simulink model "sampleModel2054_4_sub"  (R2023a)
settings: Solver=VariableStepAuto  StartTime=0.0  StopTime=10.0  RelTol=1e-3
libraries: hdlsllib x5, simulink x2
settings Model: Creator=user1  LastModifiedBy=user1

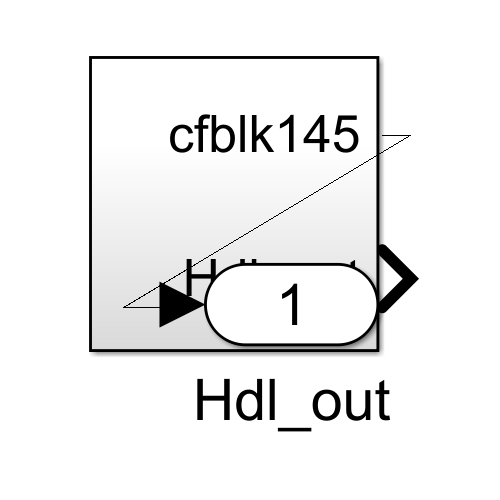
[thumbnail: Simulink's stored preview of the top-level diagram]
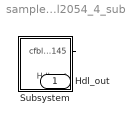
== system sampleModel2054_4_sub ==
  Subsystem : Subsystem
  Hdl_out : Outport  OutDataTypeStr=uint8
  wires:
  Subsystem/1(cfblk145) -> Hdl_out/1

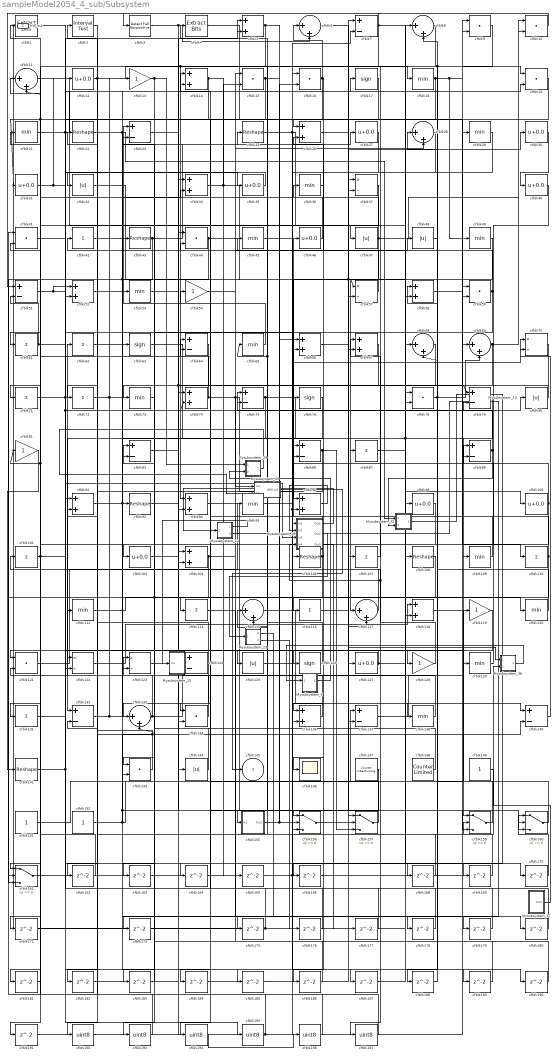
== system sampleModel2054_4_sub/Subsystem ==
  Mysubsystem_12 : Subsystem  TreatAsAtomicUnit=on  RTWFcnName=Mysubsystem_12
      settings: RTWFcnNameOpts=User specified  RTWFileNameOpts=Use function name
  Mysubsystem_13 : Subsystem  TreatAsAtomicUnit=on  RTWFcnName=Mysubsystem_13
      settings: RTWFcnNameOpts=User specified  RTWFileNameOpts=Use function name
  Mysubsystem_15 : Subsystem  TreatAsAtomicUnit=on  RTWFcnName=Mysubsystem_15
      settings: RTWFcnNameOpts=User specified  RTWFileNameOpts=Use function name
  Mysubsystem_19 : Subsystem  TreatAsAtomicUnit=on  RTWFcnName=Mysubsystem_19
      settings: RTWFcnNameOpts=User specified  RTWFileNameOpts=Use function name
  Mysubsystem_23 : Subsystem  TreatAsAtomicUnit=on  RTWFcnName=Mysubsystem_23
      settings: RTWFcnNameOpts=User specified  RTWFileNameOpts=Use function name
  Mysubsystem_24 : Subsystem  TreatAsAtomicUnit=on  RTWFcnName=Mysubsystem_24
      settings: RTWFcnNameOpts=User specified  RTWFileNameOpts=Use function name
  Mysubsystem_25 : Subsystem  TreatAsAtomicUnit=on  RTWFcnName=Mysubsystem_25
      settings: RTWFcnNameOpts=User specified  RTWFileNameOpts=Use function name
  Mysubsystem_32 : Subsystem  TreatAsAtomicUnit=on  RTWFcnName=Mysubsystem_32
      settings: RTWFcnNameOpts=User specified  RTWFileNameOpts=Use function name
  Mysubsystem_36 : Subsystem  TreatAsAtomicUnit=on  RTWFcnName=Mysubsystem_36
      settings: RTWFcnNameOpts=User specified  RTWFileNameOpts=Use function name
  Mysubsystem_37 : Subsystem  TreatAsAtomicUnit=on  RTWFcnName=Mysubsystem_37
      settings: RTWFcnNameOpts=User specified  RTWFileNameOpts=Use function name
  Mysubsystem_6 : Subsystem  TreatAsAtomicUnit=on  RTWFcnName=Mysubsystem_6
      settings: RTWFcnNameOpts=User specified  RTWFileNameOpts=Use function name
  cfblk1 : simulink/Logic and Bit Operations/Extract Bits  bitsToExtract=Upper half  numBits=8  bitIdxRange=[0 7]  outScalingMode=Preserve fixed-point scaling
      settings: LibrarySourceBlock=|
      | hdlsllib/Logic and Bit
      | Operations/Extract Bits
  cfblk{9..10,15..16,20,41,44,59,78,121,134,143} (12 alike) : DotProduct  OutDataTypeStr=uint8
  cfblk{12,27,30..31,35,40,46,98,100,103,127} (11 alike) : Bias  Bias=0.0  SaturateOnIntegerOverflow=off
  cfblk{42,61..62,71..72,87,101,107,110,114,116,131} (12 alike) : Sum  Inputs=+  OutDataTypeStr=uint8
  cfblk{5,14,26,34,52,58,66..67,74,92,94,96,104,118,136} (15 alike) : Sum  OutDataTypeStr=uint8
  cfblk{22,25,43,93,106,108,141} (7 alike) : Reshape
  cfblk{18,21,29,36,45,49,53,65,73,95,109,112,120,129,138} (15 alike) : MinMax  OutDataTypeStr=uint8
  cfblk{6,8,11,28,68..69,115,117,133} (9 alike) : Sum  Inputs=|++  OutDataTypeStr=uint8
  cfblk{13,54,81,119,128} (5 alike) : Gain  OutDataTypeStr=uint8
  cfblk{37,57,70,122..123} (5 alike) : Product  Inputs=*/  OutDataTypeStr=uint8  RndMeth=Zero  SaturateOnIntegerOverflow=on
  cfblk{7,23,51,64,75,79,83,86,89,124,132,137,140} (13 alike) : Sum  Inputs=+-  OutDataTypeStr=uint8
  cfblk{32,47..48,80,125,144} (6 alike) : Abs  OutDataTypeStr=uint8  SaturateOnIntegerOverflow=off
  cfblk{17,63,76,126} (4 alike) : Signum
  cfblk146 : Scope
  cfblk147 : hdlsllib/Sources/Counter Free-Running  NumBits=16  tsamp=-1
  cfblk148 : hdlsllib/Sources/Counter Limited  uplimit=7  tsamp=-1
  cfblk149 : Constant  OutDataTypeStr=uint8  SampleTime=-1
  cfblk151 : Constant  OutDataTypeStr=uint8  SampleTime=-1
  cfblk152 : Constant  OutDataTypeStr=uint8  SampleTime=-1
  cfblk155 : Subsystem
      settings: LibrarySourceBlock=|
      | hdlsllib/Ports &
      | Subsystems/Subsystem
  cfblk{156..157,159..161} (5 alike) : Switch  OutDataTypeStr=uint8  SaturateOnIntegerOverflow=off  InputSameDT=off
  cfblk{162..166,168..171,173,175..191} (27 alike) : Delay  SampleTime=1
  cfblk{192..197} (6 alike) : DataTypeConversion  OutDataTypeStr=uint8  SaturateOnIntegerOverflow=off  RndMeth=Floor
  cfblk2 : hdlsllib/Logic and Bit Operations/Interval Test  IntervalClosedRight=on  uplimit=0.5  IntervalClosedLeft=on  lowlimit=-0.5  OutDataTypeStr=uint8
  cfblk3 : hdlsllib/Logic and Bit Operations/Detect Fall Nonpositive  vinit=0  OutDataTypeStr=uint8
  cfblk4 : simulink/Logic and Bit Operations/Extract Bits  bitsToExtract=Upper half  numBits=8  bitIdxRange=[0 7]  outScalingMode=Preserve fixed-point scaling
      settings: LibrarySourceBlock=|
      | hdlsllib/Logic and Bit
      | Operations/Extract Bits
  cfblk145 : Outport  OutDataTypeStr=uint8  VectorParamsAs1DForOutWhenUnconnected=off
  Hdl_out : Outport  Port=2  OutDataTypeStr=uint8
  wires:
  cfblk5/1 -> cfblk66/1, cfblk61/1, cfblk94/1
  cfblk127/1 -> cfblk80/1, cfblk121/1
  cfblk79/1 -> cfblk159/1
  cfblk72/1 -> cfblk190/1, cfblk63/1
  cfblk51/1 -> cfblk170/1, cfblk52/1
  cfblk94/1 -> cfblk156/1
  cfblk70/1 -> cfblk114/1
  cfblk43/1 -> cfblk161/2, cfblk25/1
  cfblk144/1 -> cfblk83/1
  cfblk15/1 -> cfblk156/2, cfblk191/1, cfblk31/1
  cfblk86/1 -> cfblk162/1, cfblk157/3
  cfblk76/1 -> cfblk132/1
  cfblk57/1 -> cfblk42/1
  cfblk110/1 -> cfblk122/2, cfblk46/1
  cfblk41/1 -> cfblk195/1
  cfblk122/1 -> cfblk118/1
  cfblk81/1 -> cfblk141/1
  cfblk62/1 -> cfblk27/1
  cfblk117/1 -> cfblk64/1
  cfblk65/1 -> cfblk23/1
  cfblk44/1 -> cfblk183/1, cfblk57/2, cfblk98/1
  cfblk49/1 -> cfblk96/1
  cfblk59/1 -> cfblk36/1, cfblk133/1
  cfblk16/1 -> cfblk182/1, cfblk146/1, cfblk6/1
  cfblk10/1 -> cfblk51/1
  cfblk3/1 -> cfblk117/2, cfblk6/2
  cfblk30/1 -> cfblk40/1
  cfblk148/1 -> cfblk53/1
  cfblk149/1 -> cfblk159/2
  cfblk13/1 -> cfblk133/2, Mysubsystem_24/1(In1)
  cfblk20/1 -> cfblk125/1
  cfblk63/1 -> cfblk108/1
  cfblk45/1 -> cfblk47/1
  cfblk112/1 -> cfblk120/1
  cfblk151/1 -> cfblk137/1
  cfblk78/1 -> cfblk178/1, cfblk69/2
  cfblk34/1 -> cfblk15/2, cfblk117/1
  cfblk83/1 -> cfblk124/1
  cfblk161/1 -> cfblk37/2, cfblk16/1
  cfblk136/1 -> cfblk62/1
  cfblk32/1 -> cfblk127/1
  cfblk42/1 -> cfblk168/1, cfblk160/2
  cfblk61/1 -> cfblk20/2, cfblk51/2
  cfblk52/1 -> cfblk87/1
  cfblk126/1 -> cfblk4/1
  cfblk159/1 -> cfblk119/1
  cfblk25/1 -> cfblk140/1, cfblk78/1
  cfblk95/1 -> cfblk7/2
  cfblk98/1 -> cfblk155/1(In1)
  cfblk128/1 -> Mysubsystem_19/4(In4), cfblk101/1
  cfblk106/1 -> cfblk44/2, cfblk143/1
  cfblk26/1 -> cfblk159/3
  cfblk73/1 -> cfblk43/1
  cfblk11/1 -> cfblk78/2
  cfblk121/1 -> cfblk95/1
  cfblk119/1 -> cfblk131/1
  cfblk8/1 -> cfblk115/2
  cfblk74/1 -> cfblk21/1, cfblk106/1, Mysubsystem_25/1(In1)
  cfblk160/1 -> cfblk58/1
  cfblk18/1 -> cfblk71/1, cfblk20/1, cfblk49/1
  cfblk138/1 -> cfblk75/1
  cfblk64/1 -> cfblk104/2
  cfblk157/1 -> cfblk54/1
  cfblk53/1 -> cfblk160/3, cfblk79/1
  cfblk31/1 -> cfblk189/1, cfblk12/1
  cfblk22/1 -> cfblk179/1, cfblk57/1, Mysubsystem_32/1(In1)
  cfblk47/1 -> cfblk26/2, cfblk126/1, cfblk10/1
  cfblk124/1 -> cfblk163/1, cfblk92/2
  cfblk75/1 -> cfblk134/1, cfblk107/1
  cfblk134/1 -> cfblk123/1
  cfblk116/1 -> cfblk128/1
  cfblk118/1 -> cfblk29/1
  cfblk104/1 -> cfblk48/1, cfblk193/1, cfblk161/3
  cfblk101/1 -> cfblk171/1, Mysubsystem_19/3(In3)
  cfblk100/1 -> cfblk161/1, cfblk86/2
  cfblk132/1 -> cfblk13/1, cfblk34/2
  cfblk27/1 -> cfblk137/2
  cfblk155/1(Out1) -> cfblk16/2, cfblk70/1
  cfblk129/1 -> cfblk89/1
  cfblk21/1 -> cfblk66/2, cfblk26/1, cfblk17/1
  cfblk152/1 -> cfblk140/2, cfblk59/1
  cfblk89/1 -> cfblk75/2, Mysubsystem_32/2(In2)
  cfblk103/1 -> cfblk76/1
  cfblk4/1 -> cfblk59/2
  cfblk29/1 -> cfblk96/2, Mysubsystem_19/1(In1)
  cfblk137/1 -> cfblk9/1
  cfblk69/1 -> cfblk116/1, cfblk10/2
  cfblk54/1 -> cfblk28/2
  cfblk40/1 -> cfblk109/1
  cfblk12/1 -> cfblk18/1, cfblk72/1
  cfblk156/1 -> cfblk30/1
  cfblk93/1 -> cfblk79/2
  cfblk120/1 -> cfblk8/2
  cfblk23/1 -> cfblk74/1
  cfblk35/1 -> cfblk32/1
  cfblk68/1 -> cfblk103/1
  cfblk80/1 -> cfblk73/1
  cfblk1/1 -> cfblk35/1
  cfblk9/1 -> cfblk197/1, cfblk68/2
  cfblk14/1 -> cfblk165/1, cfblk112/1
  cfblk133/1 -> cfblk118/2, cfblk81/1, cfblk11/2
  cfblk46/1 -> cfblk11/1
  cfblk67/1 -> cfblk123/2
  cfblk143/1 -> cfblk122/1, cfblk22/1
  cfblk107/1 -> cfblk67/1
  cfblk71/1 -> cfblk5/2, cfblk74/2, cfblk129/1
  cfblk58/1 -> cfblk110/1
  cfblk109/1 -> cfblk45/1, cfblk65/1
  cfblk115/1 -> cfblk138/1
  cfblk140/1 -> cfblk70/2
  cfblk28/1 -> cfblk136/1
  cfblk7/1 -> cfblk3/1, cfblk134/2, cfblk89/2, cfblk100/1
  cfblk92/1 -> cfblk14/1, cfblk93/1
  cfblk6/1 -> cfblk37/1
  cfblk141/1 -> cfblk185/1, cfblk52/2
  cfblk108/1 -> cfblk143/2
  cfblk123/1 -> cfblk5/1
  cfblk162/1 -> cfblk1/1
  cfblk163/1 -> cfblk86/1
  cfblk131/1 -> cfblk164/1
  cfblk164/1 -> cfblk157/2
  cfblk165/1 -> cfblk9/2
  cfblk166/1 -> cfblk68/1
  cfblk168/1 -> cfblk115/1
  cfblk87/1 -> cfblk169/1
  cfblk169/1 -> cfblk132/2
  cfblk170/1 -> cfblk160/1
  cfblk171/1 -> cfblk58/2
  cfblk173/1 -> cfblk156/3
  cfblk175/1 -> Hdl_out/1, cfblk64/2
  cfblk176/1 -> cfblk124/2
  cfblk177/1 -> cfblk104/1
  cfblk178/1 -> cfblk92/1
  cfblk179/1 -> cfblk14/2
  cfblk114/1 -> cfblk180/1
  cfblk180/1 -> cfblk7/1
  cfblk37/1 -> cfblk181/1
  cfblk181/1 -> cfblk121/2
  cfblk182/1 -> cfblk94/2
  cfblk183/1 -> cfblk23/2
  cfblk17/1 -> cfblk184/1
  cfblk184/1 -> cfblk157/1
  cfblk185/1 -> cfblk67/2
  cfblk36/1 -> cfblk186/1
  cfblk186/1 -> cfblk83/2
  cfblk125/1 -> cfblk187/1
  cfblk187/1 -> cfblk8/1
  cfblk48/1 -> cfblk188/1
  cfblk188/1 -> cfblk28/1
  cfblk189/1 -> cfblk34/1
  cfblk190/1 -> cfblk15/1
  cfblk191/1 -> cfblk136/2
  cfblk2/1 -> cfblk192/1
  cfblk192/1 -> cfblk144/1
  cfblk193/1 -> cfblk2/1
  cfblk147/1 -> cfblk194/1
  cfblk195/1 -> cfblk69/1, cfblk44/1
  cfblk194/1 -> cfblk196/1
  cfblk196/1 -> cfblk41/1
  cfblk197/1 -> cfblk41/2
  Mysubsystem_12/2(Out2) -> Mysubsystem_13/2(In2)
  Mysubsystem_13/1(Out1) -> cfblk166/1
  Mysubsystem_13/2(Out2) -> cfblk173/1
  Mysubsystem_12/1(Out1) -> Mysubsystem_15/1(In1)
  cfblk96/1 -> Mysubsystem_19/2(In2)
  Mysubsystem_19/1(Out1) -> Mysubsystem_12/1(In1)
  Mysubsystem_19/3(Out3) -> cfblk177/1
  Mysubsystem_19/2(Out2) -> Mysubsystem_23/1(In1)
  Mysubsystem_23/1(Out1) -> cfblk175/1
  Mysubsystem_23/2(Out2) -> cfblk176/1
  Mysubsystem_6/1(Out1) -> Mysubsystem_24/2(In2)
  Mysubsystem_24/1(Out1) -> Mysubsystem_25/2(In2)
  Mysubsystem_25/1(cfblk145) -> cfblk145/1
  Mysubsystem_32/1(Out1) -> Mysubsystem_13/1(In1)
  cfblk66/1 -> Mysubsystem_36/1(In1)
  Mysubsystem_36/1(Out1) -> Mysubsystem_6/1(In1)
  Mysubsystem_37/1(Out1) -> Mysubsystem_36/2(In2)

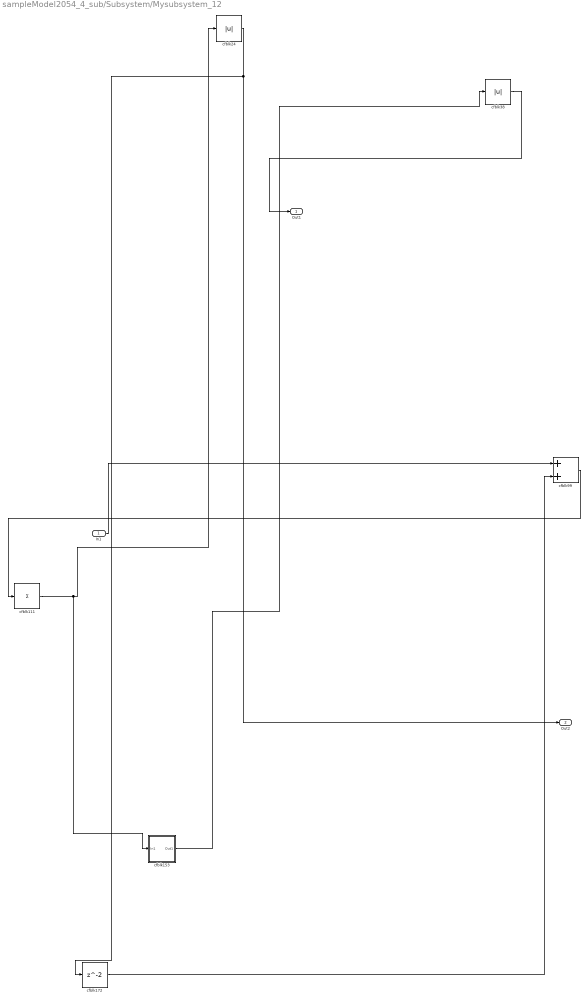
== system sampleModel2054_4_sub/Subsystem/Mysubsystem_12 ==
  In1 : Inport
  cfblk111 : Sum  Inputs=+
  cfblk153 : Subsystem
      settings: LibrarySourceBlock=|
      | hdlsllib/Ports &
      | Subsystems/Subsystem
  cfblk172 : Delay  SampleTime=1
  cfblk24 : Abs  SaturateOnIntegerOverflow=off
  cfblk38 : Abs  SaturateOnIntegerOverflow=off
  cfblk99 : Sum
  Out1 : Outport
  Out2 : Outport  Port=2
  wires:
  cfblk38/1 -> Out1/1
  cfblk153/1(Out1) -> cfblk38/1
  cfblk99/1 -> cfblk111/1
  In1/1 -> cfblk99/1
  cfblk172/1 -> cfblk99/2
  cfblk111/1 -> cfblk153/1(In1), cfblk24/1
  cfblk24/1 -> cfblk172/1, Out2/1

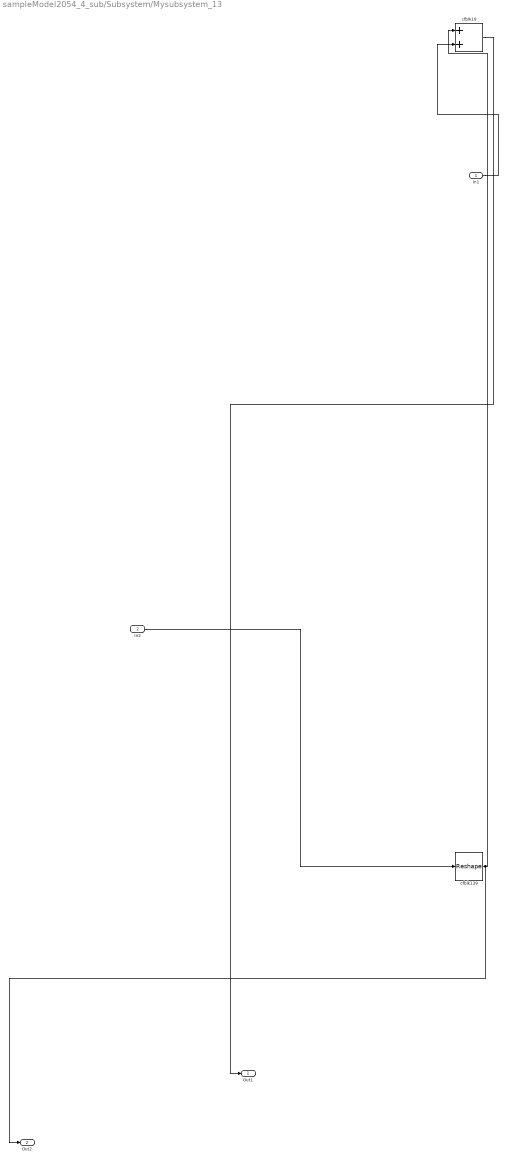
== system sampleModel2054_4_sub/Subsystem/Mysubsystem_13 ==
  In1 : Inport
  In2 : Inport  Port=2
  cfblk139 : Reshape
  cfblk19 : Sum
  Out1 : Outport
  Out2 : Outport  Port=2
  wires:
  In2/1 -> cfblk139/1
  cfblk19/1 -> Out1/1
  cfblk139/1 -> cfblk19/1, Out2/1
  In1/1 -> cfblk19/2

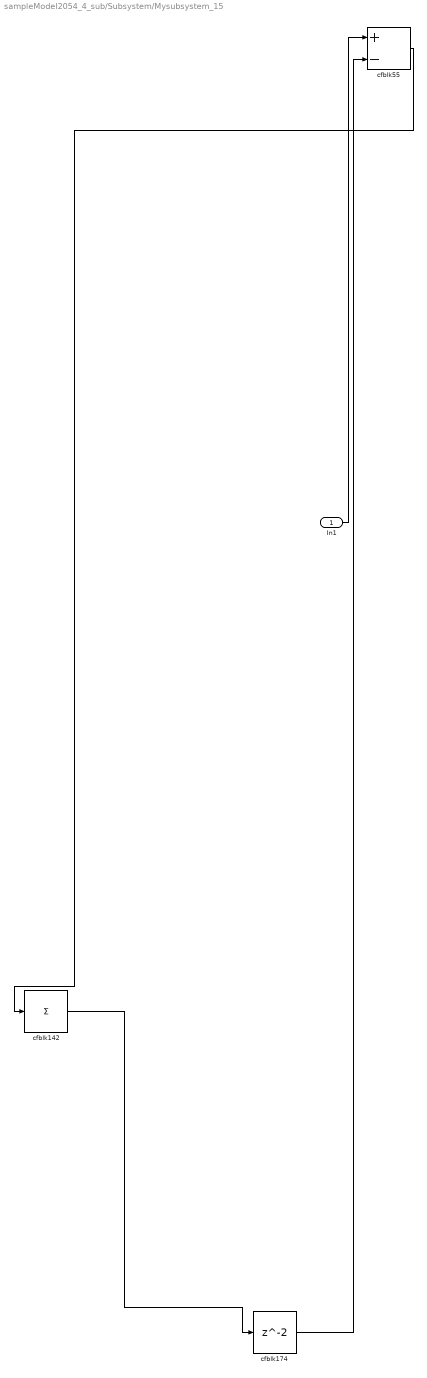
== system sampleModel2054_4_sub/Subsystem/Mysubsystem_15 ==
  In1 : Inport
  cfblk142 : Sum  Inputs=+
  cfblk174 : Delay  SampleTime=1
  cfblk55 : Sum  Inputs=+-
  wires:
  cfblk174/1 -> cfblk55/2
  cfblk142/1 -> cfblk174/1
  cfblk55/1 -> cfblk142/1
  In1/1 -> cfblk55/1

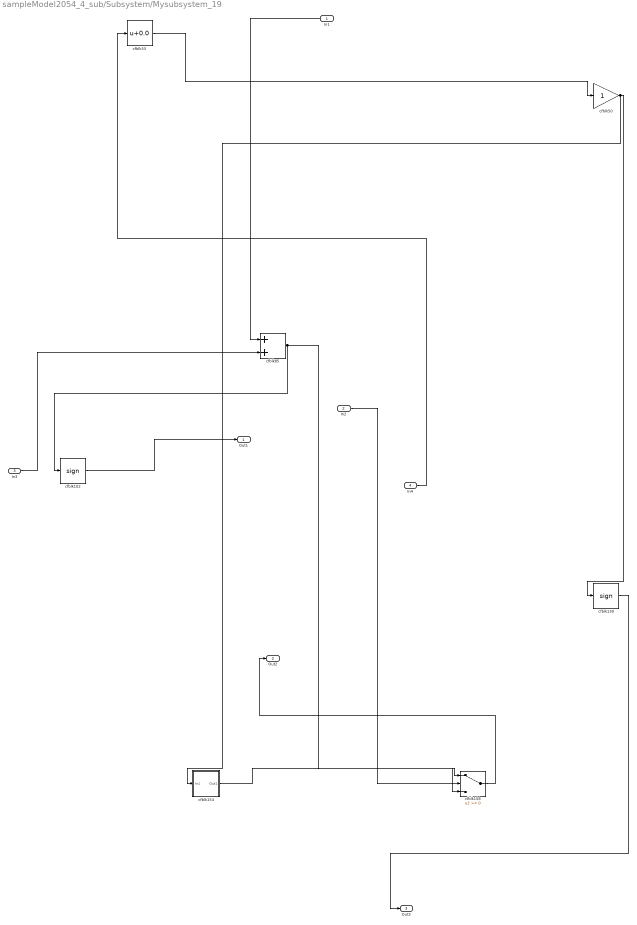
== system sampleModel2054_4_sub/Subsystem/Mysubsystem_19 ==
  In1 : Inport
  In2 : Inport  Port=2
  In3 : Inport  Port=3
  In4 : Inport  Port=4
  cfblk102 : Signum
  cfblk130 : Signum
  cfblk154 : Subsystem
      settings: LibrarySourceBlock=|
      | hdlsllib/Ports &
      | Subsystems/Subsystem
  cfblk158 : Switch  SaturateOnIntegerOverflow=off  InputSameDT=off
  cfblk33 : Bias  Bias=0.0  SaturateOnIntegerOverflow=off
  cfblk50 : Gain
  cfblk85 : Sum
  Out1 : Outport
  Out2 : Outport  Port=2
  Out3 : Outport  Port=3
  wires:
  cfblk102/1 -> Out1/1
  In4/1 -> cfblk33/1
  cfblk158/1 -> Out2/1
  In1/1 -> cfblk85/1
  In2/1 -> cfblk158/2
  In3/1 -> cfblk85/2
  cfblk130/1 -> Out3/1
  cfblk85/1 -> cfblk158/3, cfblk102/1
  cfblk33/1 -> cfblk50/1
  cfblk50/1 -> cfblk130/1, cfblk154/1(In1)
  cfblk154/1(Out1) -> cfblk158/1

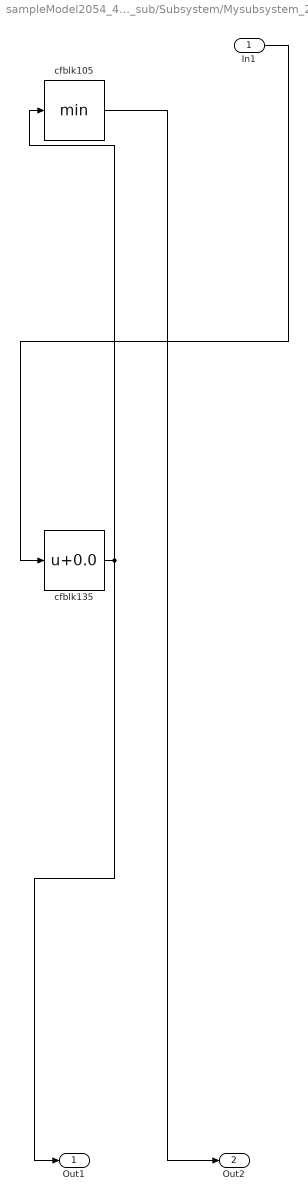
== system sampleModel2054_4_sub/Subsystem/Mysubsystem_23 ==
  In1 : Inport
  cfblk105 : MinMax
  cfblk135 : Bias  Bias=0.0  SaturateOnIntegerOverflow=off
  Out1 : Outport
  Out2 : Outport  Port=2
  wires:
  cfblk105/1 -> Out2/1
  In1/1 -> cfblk135/1
  cfblk135/1 -> cfblk105/1, Out1/1

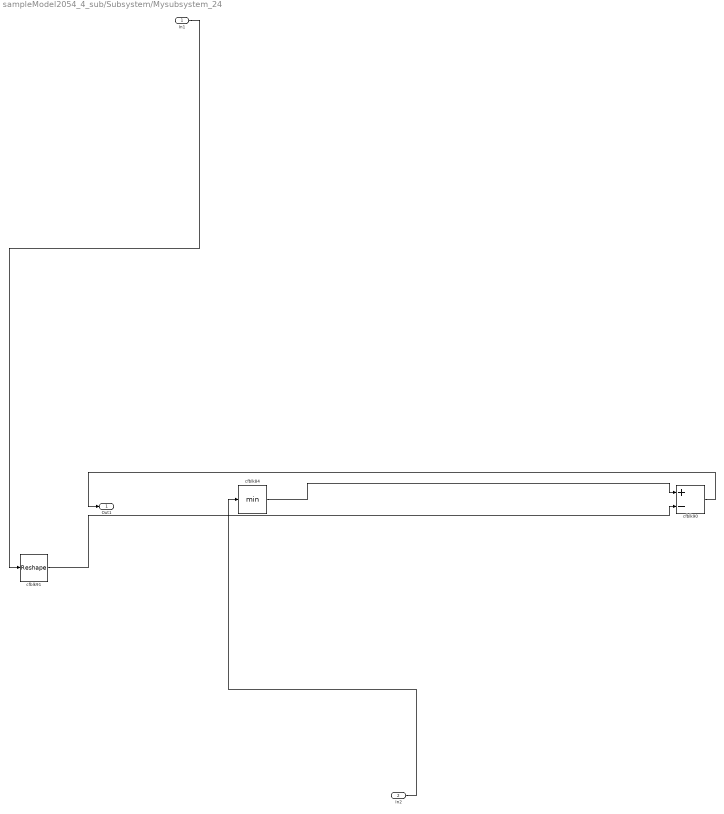
== system sampleModel2054_4_sub/Subsystem/Mysubsystem_24 ==
  In1 : Inport
  In2 : Inport  Port=2
  cfblk84 : MinMax
  cfblk90 : Sum  Inputs=+-
  cfblk91 : Reshape
  Out1 : Outport
  wires:
  In2/1 -> cfblk84/1
  cfblk84/1 -> cfblk90/1
  cfblk90/1 -> Out1/1
  cfblk91/1 -> cfblk90/2
  In1/1 -> cfblk91/1

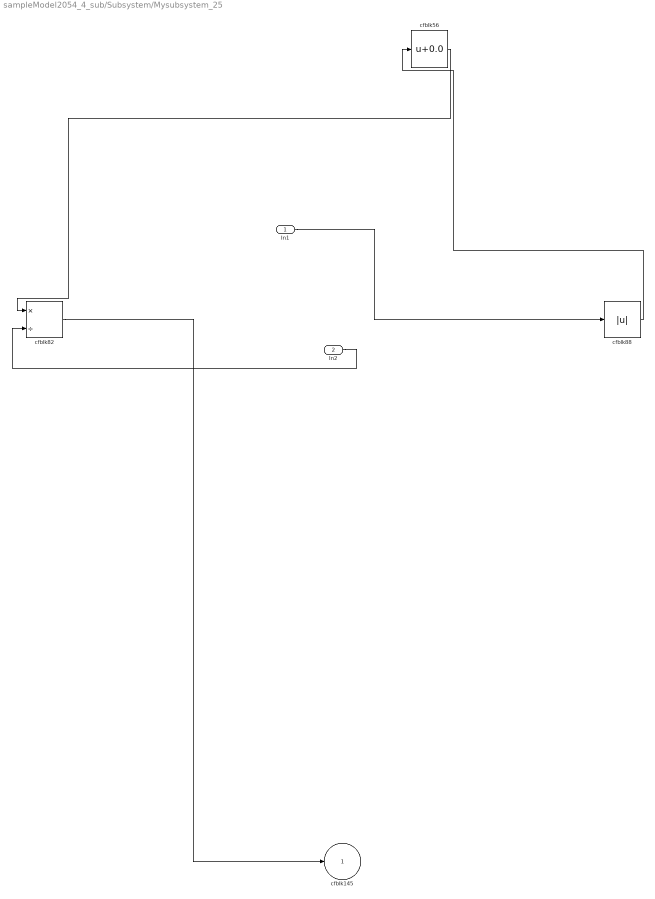
== system sampleModel2054_4_sub/Subsystem/Mysubsystem_25 ==
  In1 : Inport
  In2 : Inport  Port=2
  cfblk56 : Bias  Bias=0.0  SaturateOnIntegerOverflow=off
  cfblk82 : Product  Inputs=*/  RndMeth=Zero  SaturateOnIntegerOverflow=on
  cfblk88 : Abs  SaturateOnIntegerOverflow=off
  cfblk145 : Outport  VectorParamsAs1DForOutWhenUnconnected=off
  wires:
  In2/1 -> cfblk82/2
  cfblk88/1 -> cfblk56/1
  In1/1 -> cfblk88/1
  cfblk56/1 -> cfblk82/1
  cfblk82/1 -> cfblk145/1

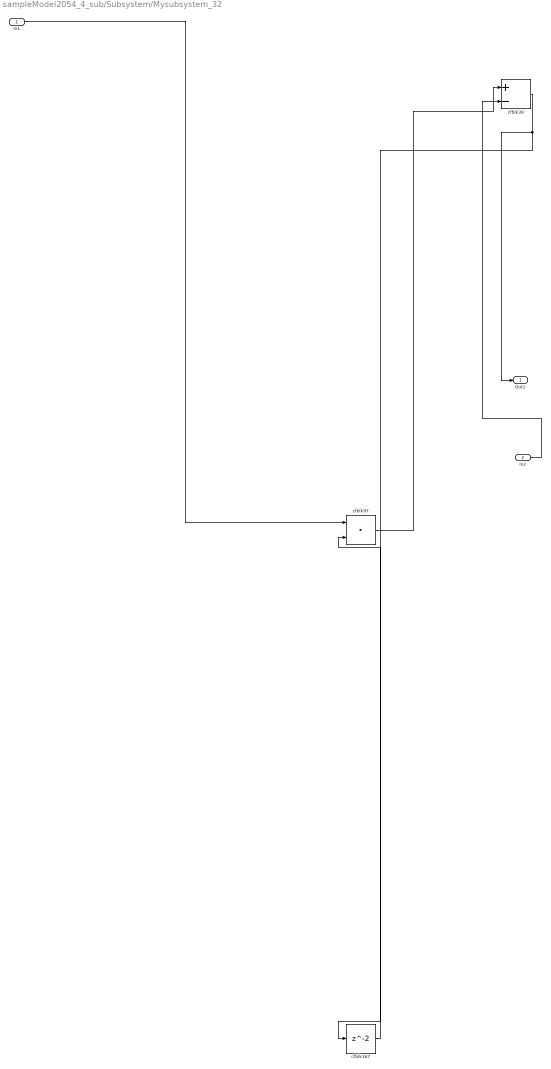
== system sampleModel2054_4_sub/Subsystem/Mysubsystem_32 ==
  In1 : Inport
  In2 : Inport  Port=2
  cfblk167 : Delay  SampleTime=1
  cfblk39 : Sum  Inputs=+-
  cfblk97 : DotProduct  OutDataTypeStr=Inherit: Inherit via internal rule
  Out1 : Outport
  wires:
  In2/1 -> cfblk39/2
  cfblk97/1 -> cfblk39/1
  cfblk167/1 -> cfblk97/2
  cfblk39/1 -> cfblk167/1, Out1/1
  In1/1 -> cfblk97/1

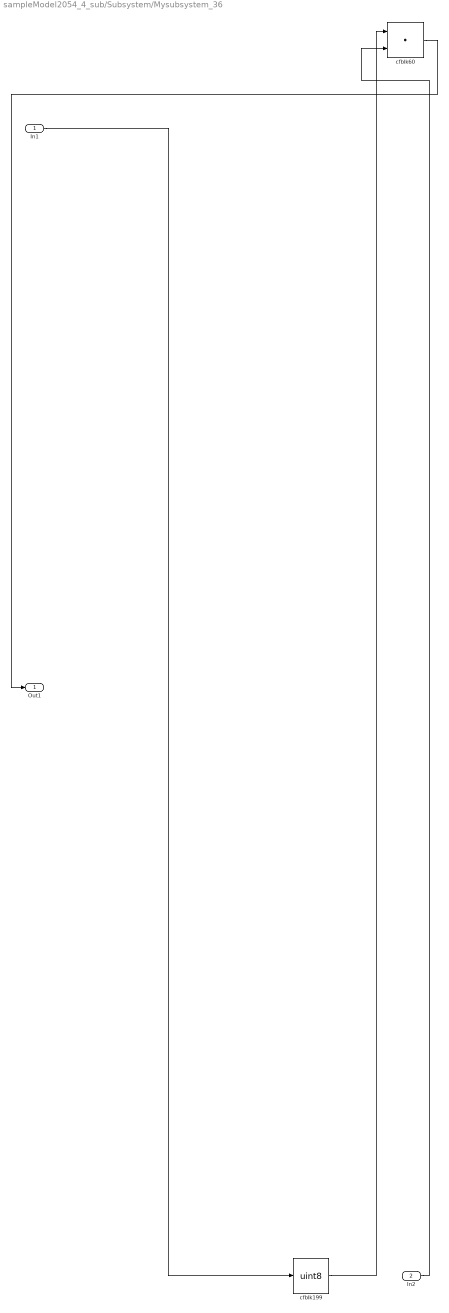
== system sampleModel2054_4_sub/Subsystem/Mysubsystem_36 ==
  In1 : Inport
  In2 : Inport  Port=2
  cfblk199 : DataTypeConversion  OutDataTypeStr=uint8  SaturateOnIntegerOverflow=off  RndMeth=Floor
  cfblk60 : DotProduct  OutDataTypeStr=Inherit: Inherit via internal rule
  Out1 : Outport
  wires:
  cfblk60/1 -> Out1/1
  In1/1 -> cfblk199/1
  cfblk199/1 -> cfblk60/1
  In2/1 -> cfblk60/2

== system sampleModel2054_4_sub/Subsystem/Mysubsystem_37 ==
  cfblk150 : hdlsllib/Sources/Counter Limited  uplimit=7  tsamp=-1
  cfblk200 : DataTypeConversion  OutDataTypeStr=uint8  SaturateOnIntegerOverflow=off  RndMeth=Floor
  Out1 : Outport
  wires:
  cfblk200/1 -> Out1/1
  cfblk150/1 -> cfblk200/1

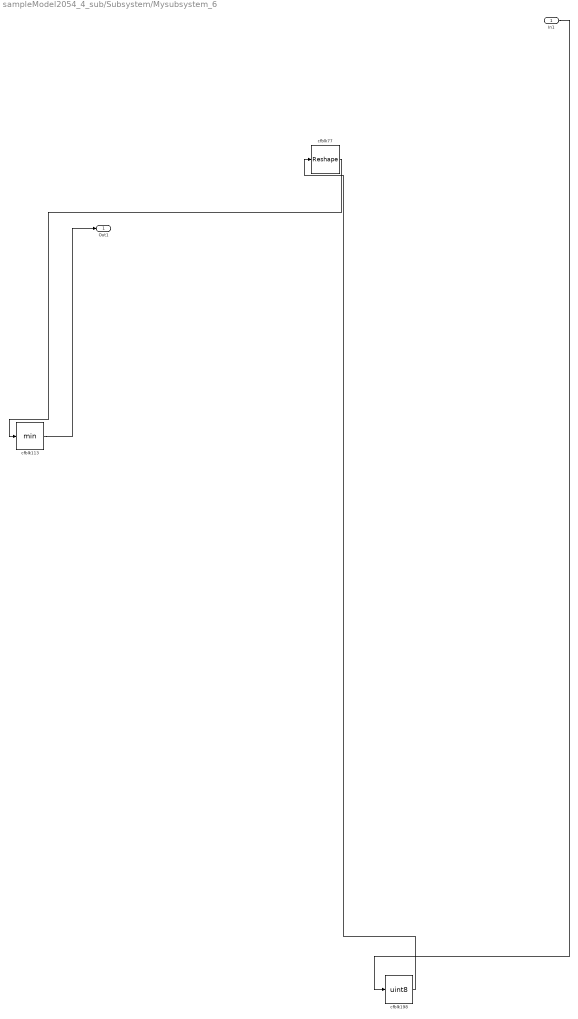
== system sampleModel2054_4_sub/Subsystem/Mysubsystem_6 ==
  In1 : Inport
  cfblk113 : MinMax
  cfblk198 : DataTypeConversion  OutDataTypeStr=uint8  SaturateOnIntegerOverflow=off  RndMeth=Floor
  cfblk77 : Reshape
  Out1 : Outport
  wires:
  In1/1 -> cfblk198/1
  cfblk113/1 -> Out1/1
  cfblk198/1 -> cfblk77/1
  cfblk77/1 -> cfblk113/1

== system sampleModel2054_4_sub/Subsystem/cfblk155 ==
  In1 : Inport
  Out1 : Outport
  wires:
  In1/1 -> Out1/1

== system sampleModel2054_4_sub/Subsystem/Mysubsystem_12/cfblk153 ==
  In1 : Inport
  Out1 : Outport
  wires:
  In1/1 -> Out1/1

== system sampleModel2054_4_sub/Subsystem/Mysubsystem_19/cfblk154 ==
  In1 : Inport
  Out1 : Outport
  wires:
  In1/1 -> Out1/1
